simulink model "gm_sampleModel12940_sub"  (R2023b)
settings: Solver=VariableStepAuto  StartTime=0.0  StopTime=10.0  RelTol=1e-3
libraries: hdlsllib x3, simulink x2
(part 1 of 2)
settings Model: Creator=Tsmc  LastModifiedBy=Tsmc
settings OptimizationCC: BlockReduction=off  ConditionallyExecuteInputs=off
settings DebuggingCC: InheritedTsInSrcMsg=none

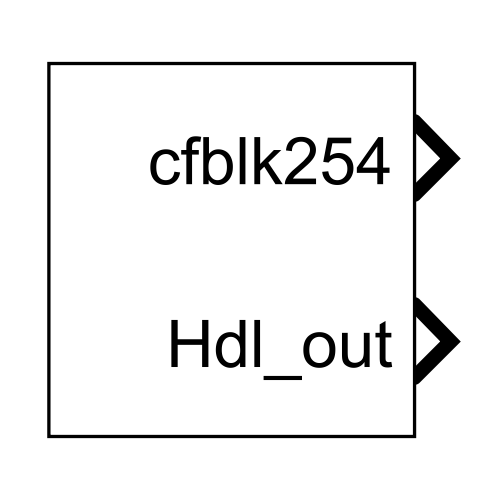
[thumbnail: Simulink's stored preview of the top-level diagram]
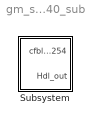
== system gm_sampleModel12940_sub ==
  Subsystem : Subsystem

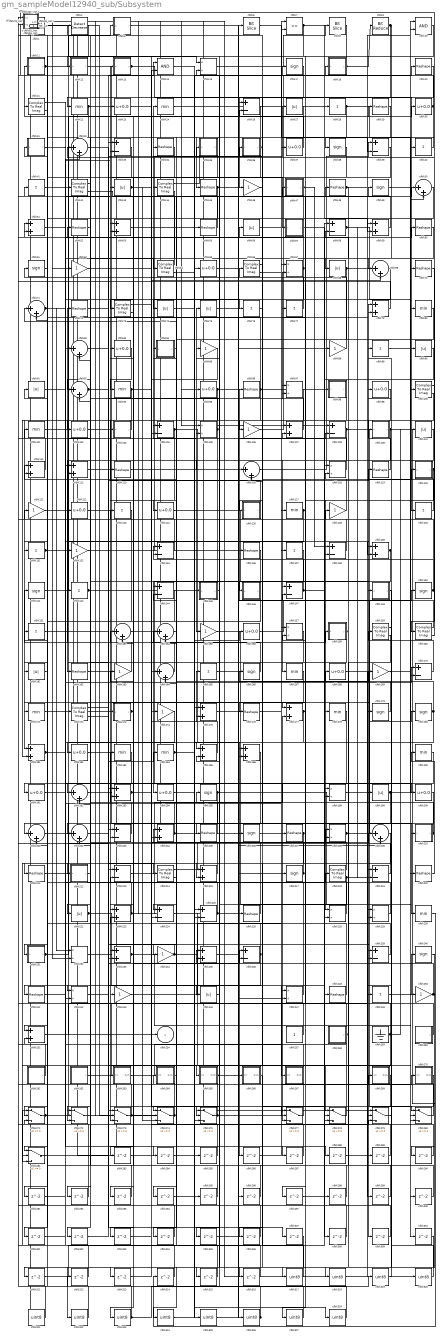
== system gm_sampleModel12940_sub/Subsystem ==
  cfblk1 : simulink/Logic and Bit Operations/Detect Decrease  vinit=0.0  OutDataTypeStr=uint8
      settings: LibrarySourceBlock=|
      | hdlsllib/Logic and Bit
      | Operations/Detect
      | Decrease
  cfblk10 : Logic  AllPortsSameDT=off  OutDataTypeStr=boolean
  cfblk{21,42,44,64,66,73,100,159..160,172,214,218} (12 alike) : ComplexToRealImag
  cfblk100_term0 : Terminator
  cfblk{22,24,80,93,101,127,167,171,178,183..184,190,230} (13 alike) : MinMax  OutDataTypeStr=uint8
  cfblk{23,30,37,65,83,95,99,102,122,124,156,168,182,191,194,200} (16 alike) : Bias  Bias=0.0  SaturateOnIntegerOverflow=off
  cfblk103 : Subsystem  mask(Real World Value Increment){}
      mask help: Simulink:masks:RealWorldValueIncrement_MD
      mask Display: disp('V++')
  cfblk{26,33,39,58,104,108,134,138,144,147,170,203,213,219,224..225,236,239} (18 alike) : Sum  Inputs=+-  OutDataTypeStr=uint8
  cfblk{15,67,97,105,118,157,198,208,228..229,232,242,247} (13 alike) : Product  Inputs=*/  OutDataTypeStr=uint8  RndMeth=Zero  SaturateOnIntegerOverflow=on
  cfblk{46,62,85,88,106,121,128,132,155,163,169,174,234,243,250} (15 alike) : Gain  OutDataTypeStr=uint8
  cfblk{51,53,59,79,107,111..112,139,175,177,181,185..186,193,204,215,223,233,235,251} (20 alike) : Sum  OutDataTypeStr=uint8
  cfblk109 : Subsystem  mask(Real World Value Increment){}
      mask help: Simulink:masks:RealWorldValueIncrement_MD
      mask Display: disp('V++')
  cfblk11 : Subsystem  mask(Compare To Zero){relop=<=, OutDataTypeStr=uint8, ZeroCross=on}
      mask prompts: relop "Simulink:masks:Operator_MP"; OutDataTypeStr "Simulink:masks:OutputDataType_MP"; ZeroCross "Simulink:masks:EnableZerocrossingDetection_MP"
      mask help: Simulink:masks:CompareToZero_MD
      mask init:
      | OutDataTypeStr = 'uint8';
      | ZeroCross = 'on';
      | blkName = 'sampleModel12940_sub/Subsystem/cfblk11';
      | relop = '<=';
      | setValue = 'fixdt(0, 8)';
      mask TypeOptions relop: == | ~= | < | <= | >= | >
      mask TypeOptions OutDataTypeStr: Simulink:masks:uint8 | Simulink:masks:boolean
      mask Callback ZeroCross: sl('zeroCrossEnable', gcbh);
      mask Display: disp([relop,' 0'])
  cfblk{27,43,56,68,74..75,90..91,110,161,199,222,245} (13 alike) : Abs  OutDataTypeStr=uint8  SaturateOnIntegerOverflow=off
  cfblk{20,29,34,45,48,52,55,60,70,72,96,113,119,136,162,176,205,207,211,220,226,241,248} (23 alike) : Reshape
  cfblk115_inst : Subsystem
  cfblk{32,50,69,71,82,92,116,153..154,164,192,201..202,209} (14 alike) : Sum  Inputs=|++  OutDataTypeStr=uint8
  cfblk12 : Subsystem  mask(Detect Rise Positive){vinit=double(0), InputProcessing=Elements as channels (sample based), OutDataTypeStr=uint8}
      mask prompts: vinit "Simulink:masks:InitialCondition_MP"; InputProcessing "Simulink:masks:InputProcessing_MP"; OutDataTypeStr "Simulink:masks:OutputDataType_MP"
      mask help: Simulink:masks:DetectRisePositive_MD
      mask init:
      | InputProcessing = 'Elements as channels (sample based)';
      | OutDataTypeStr = 'uint8';
      | vinit = double(0);
      mask TypeOptions InputProcessing: Simulink:masks:ColumnsAsChannelsFrameBased | Simulink:masks:ElementsAsChannelsSampleBased
      mask TypeOptions OutDataTypeStr: Simulink:masks:uint8 | Simulink:masks:boolean
      mask Display: fprintf('U > 0\n&  NOT\nU/z > 0')
  cfblk120 : Subsystem  mask(Real World Value Increment){}
      mask help: Simulink:masks:RealWorldValueIncrement_MD
      mask Display: disp('V++')
  cfblk{28,40..41,76..77,89,123,130..131,137,142,151,165,249} (14 alike) : Sum  Inputs=+  OutDataTypeStr=uint8
  cfblk126 : Subsystem  mask(Real World Value Increment){}
      mask help: Simulink:masks:RealWorldValueIncrement_MD
      mask Display: disp('V++')
  cfblk129_inst : Subsystem
  cfblk13 : Subsystem  mask(Compare To Zero){relop=<=, OutDataTypeStr=uint8, ZeroCross=on}
      mask prompts: relop "Simulink:masks:Operator_MP"; OutDataTypeStr "Simulink:masks:OutputDataType_MP"; ZeroCross "Simulink:masks:EnableZerocrossingDetection_MP"
      mask help: Simulink:masks:CompareToZero_MD
      mask init:
      | OutDataTypeStr = 'uint8';
      | ZeroCross = 'on';
      | blkName = 'sampleModel12940_sub/Subsystem/cfblk13';
      | relop = '<=';
      | setValue = 'fixdt(0, 8)';
      mask TypeOptions relop: == | ~= | < | <= | >= | >
      mask TypeOptions OutDataTypeStr: Simulink:masks:uint8 | Simulink:masks:boolean
      mask Callback ZeroCross: sl('zeroCrossEnable', gcbh);
      mask Display: disp([relop,' 0'])
  cfblk14 : Logic  AllPortsSameDT=off  OutDataTypeStr=boolean
  cfblk{17,38,49,61,141,150,166,179..180,195,206,217,240} (13 alike) : Signum
  cfblk145 : Subsystem  mask(Real World Value Increment){}
      mask help: Simulink:masks:RealWorldValueIncrement_MD
      mask Display: disp('V++')
  cfblk146 : Subsystem  mask(Real World Value Increment){}
      mask help: Simulink:masks:RealWorldValueIncrement_MD
      mask Display: disp('V++')
  cfblk148_inst : Subsystem
  cfblk149 : Subsystem  mask(Real World Value Increment){}
      mask help: Simulink:masks:RealWorldValueIncrement_MD
      mask Display: disp('V++')
  cfblk152_inst : Subsystem
  cfblk158 : Subsystem  mask(Real World Value Increment){}
      mask help: Simulink:masks:RealWorldValueIncrement_MD
      mask Display: disp('V++')
  cfblk16_inst : Subsystem
  cfblk173 : Subsystem  mask(Real World Value Increment){}
      mask help: Simulink:masks:RealWorldValueIncrement_MD
      mask Display: disp('V++')
  cfblk18 : Subsystem  mask(Real World Value Increment){}
      mask help: Simulink:masks:RealWorldValueIncrement_MD
      mask Display: disp('V++')
  cfblk19_inst : Subsystem
  cfblk2 : simulink/Logic and Bit Operations/Detect Decrease  vinit=0.0  OutDataTypeStr=uint8
      settings: LibrarySourceBlock=|
      | hdlsllib/Logic and Bit
      | Operations/Detect
      | Decrease
  cfblk210 : Subsystem  mask(Real World Value Increment){}
      mask help: Simulink:masks:RealWorldValueIncrement_MD
      mask Display: disp('V++')
  cfblk212 : Subsystem  mask(Real World Value Increment){}
      mask help: Simulink:masks:RealWorldValueIncrement_MD
      mask Display: disp('V++')
  cfblk216_inst : Subsystem
  cfblk21_term1 : Terminator
  cfblk221_inst : Subsystem
  cfblk231 : Subsystem  mask(Real World Value Increment){}
      mask help: Simulink:masks:RealWorldValueIncrement_MD
      mask Display: disp('V++')
  cfblk257 : Constant  OutDataTypeStr=uint8  SampleTime=-1
  cfblk258 : Subsystem  mask(Counter Limited){uplimit=double(7), tsamp=double(-1)}
      mask prompts: uplimit "Simulink:masks:UpperLimit_MP"; tsamp "Simulink:masks:SampleTime_MP"
      mask help: Simulink:masks:CounterLimited_MD
      mask init:
      | nbits = double(8);
      | tsamp = double(-1);
      | uplimit = double(7);
  cfblk259 : Ground
  cfblk260 : Subsystem  mask(Counter Free-Running){NumBits=double(16), tsamp=double(-1)}
      mask prompts: NumBits "Simulink:masks:NumberOfBits_MP"; tsamp "Simulink:masks:SampleTime_MP"
      mask help: Simulink:masks:CounterFreeRunning_MD
  cfblk261 : Subsystem  mask(Counter Limited){uplimit=double(7), tsamp=double(-1)}
      mask prompts: uplimit "Simulink:masks:UpperLimit_MP"; tsamp "Simulink:masks:SampleTime_MP"
      mask help: Simulink:masks:CounterLimited_MD
      mask init:
      | nbits = double(8);
      | tsamp = double(-1);
      | uplimit = double(7);
  cfblk262 : Subsystem  mask(Counter Limited){uplimit=double(7), tsamp=double(-1)}
      mask prompts: uplimit "Simulink:masks:UpperLimit_MP"; tsamp "Simulink:masks:SampleTime_MP"
      mask help: Simulink:masks:CounterLimited_MD
      mask init:
      | nbits = double(8);
      | tsamp = double(-1);
      | uplimit = double(7);
  cfblk263 : Subsystem
  cfblk264 : Subsystem
  cfblk265 : Subsystem
  cfblk266 : Subsystem
  cfblk267 : Subsystem
  cfblk269 : Subsystem
  cfblk270 : Subsystem
  cfblk{271..275,277..281} (10 alike) : Switch  OutDataTypeStr=uint8  SaturateOnIntegerOverflow=off  InputSameDT=off
  cfblk{283..316} (34 alike) : Delay  SampleTime=1
  cfblk3 : Subsystem  mask(Detect Fall Nonpositive){vinit=double(0), InputProcessing=Elements as channels (sample based), OutDataTypeStr=uint8}
      mask prompts: vinit "Simulink:masks:InitialCondition_MP"; InputProcessing "Simulink:masks:InputProcessing_MP"; OutDataTypeStr "Simulink:masks:OutputDataType_MP"
      mask help: Simulink:masks:DetectFallNonpositive_MD
      mask init:
      | InputProcessing = 'Elements as channels (sample based)';
      | OutDataTypeStr = 'uint8';
      | vinit = double(0);
      mask TypeOptions InputProcessing: Simulink:masks:ColumnsAsChannelsFrameBased | Simulink:masks:ElementsAsChannelsSampleBased
      mask TypeOptions OutDataTypeStr: Simulink:masks:uint8 | Simulink:masks:boolean
      mask Display: fprintf('U <= 0\n&  NOT\nU/z <= 0')
  cfblk31 : Subsystem  mask(Real World Value Increment){}
      mask help: Simulink:masks:RealWorldValueIncrement_MD
      mask Display: disp('V++')
  cfblk{317..328} (12 alike) : DataTypeConversion  OutDataTypeStr=uint8  SaturateOnIntegerOverflow=off  RndMeth=Floor
  cfblk35 : Subsystem  mask(Real World Value Increment){}
      mask help: Simulink:masks:RealWorldValueIncrement_MD
      mask Display: disp('V++')
  cfblk36 : Subsystem  mask(Real World Value Increment){}
      mask help: Simulink:masks:RealWorldValueIncrement_MD
      mask Display: disp('V++')
  cfblk47 : Subsystem  mask(Real World Value Increment){}
      mask help: Simulink:masks:RealWorldValueIncrement_MD
      mask Display: disp('V++')
  cfblk57 : Subsystem  mask(Real World Value Increment){}
      mask help: Simulink:masks:RealWorldValueIncrement_MD
      mask Display: disp('V++')
  cfblk6 : hdlsllib/Logic and Bit Operations/Bit Slice  lidx=7  ridx=0
  cfblk63_inst : Subsystem
  cfblk7 : RelationalOperator  Operator=<=  OutDataTypeStr=boolean  InputSameDT=off
  cfblk78_inst : Subsystem
  cfblk8 : hdlsllib/Logic and Bit Operations/Bit Slice  lidx=7  ridx=0
  cfblk81_inst : Subsystem
  cfblk84 : Subsystem  mask(Real World Value Increment){}
      mask help: Simulink:masks:RealWorldValueIncrement_MD
      mask Display: disp('V++')
  cfblk9 : hdlsllib/Logic and Bit Operations/Bit Reduce  mode=AND
  cfblk94_inst : Subsystem
  cfblk98 : Subsystem  mask(Real World Value Increment){}
      mask help: Simulink:masks:RealWorldValueIncrement_MD
      mask Display: disp('V++')
  cfblk254 : Outport  OutDataTypeStr=uint8  SampleTime=1  VectorParamsAs1DForOutWhenUnconnected=off
  Hdl_out : Outport  Port=2  OutDataTypeStr=uint8  SampleTime=1
  wires:
  cfblk1/1 -> cfblk15/1
  cfblk10/1 -> cfblk273/3
  cfblk100/1 -> cfblk100_term0/1
  cfblk100/2 -> cfblk309/1
  cfblk101/1 -> cfblk185/1
  cfblk102/1 -> cfblk273/2
  cfblk103/1(y) -> cfblk181/1
  cfblk104/1 -> cfblk203/2, cfblk286/1
  cfblk105/1 -> cfblk216_inst/2(in2), cfblk194/1
  cfblk106/1 -> cfblk20/1
  cfblk107/1 -> cfblk67/2
  cfblk108/1 -> cfblk280/1, cfblk167/1
  cfblk109/1(y) -> cfblk311/1, cfblk155/1
  cfblk11/1(y) -> cfblk3/1(U), cfblk254/1
  cfblk110/1 -> cfblk162/1
  cfblk111/1 -> cfblk19_inst/1(in1)
  cfblk112/1 -> cfblk296/1
  cfblk113/1 -> cfblk75/1
  cfblk115_inst/1(out1) -> cfblk320/1
  cfblk116/1 -> cfblk39/1
  cfblk118/1 -> cfblk24/1
  cfblk119/1 -> cfblk79/1
  cfblk12/1(Y) -> cfblk277/3
  cfblk120/1(y) -> cfblk277/1, cfblk228/1, cfblk228/2, cfblk229/2
  cfblk121/1 -> cfblk273/1
  cfblk122/1 -> cfblk230/1
  cfblk123/1 -> cfblk281/1
  cfblk124/1 -> cfblk149/1(u)
  cfblk126/1(y) -> cfblk13/1(u)
  cfblk127/1 -> cfblk275/2, cfblk182/1, cfblk177/1, cfblk305/1
  cfblk128/1 -> cfblk34/1
  cfblk129_inst/1(out1) -> cfblk279/1, cfblk285/1, cfblk173/1(u)
  cfblk13/1(y) -> cfblk46/1, cfblk130/1
  cfblk130/1 -> cfblk16_inst/1(in1)
  cfblk131/1 -> cfblk26/2, cfblk172/1
  cfblk132/1 -> cfblk6/1
  cfblk134/1 -> cfblk123/1
  cfblk136/1 -> cfblk293/1
  cfblk137/1 -> cfblk283/1
  cfblk138/1 -> cfblk221_inst/1(in1)
  cfblk139/1 -> cfblk205/1, cfblk292/1
  cfblk14/1 -> cfblk295/1
  cfblk141/1 -> cfblk105/2
  cfblk142/1 -> cfblk82/2, cfblk147/1, cfblk229/1
  cfblk144/1 -> cfblk271/2
  cfblk145/1(y) -> cfblk95/1
  cfblk146/1(y) -> cfblk302/1
  cfblk147/1 -> cfblk278/3, cfblk85/1
  cfblk148_inst/1(out1) -> cfblk98/1(u)
  cfblk149/1(y) -> cfblk249/1
  cfblk15/1 -> cfblk8/1
  cfblk150/1 -> cfblk134/1, cfblk128/1
  cfblk151/1 -> cfblk213/1
  cfblk152_inst/1(out1) -> cfblk226/1, cfblk232/2
  cfblk153/1 -> cfblk247/1
  cfblk154/1 -> cfblk84/1(u)
  cfblk155/1 -> cfblk310/1
  cfblk156/1 -> cfblk100/1
  cfblk157/1 -> cfblk303/1
  cfblk158/1(y) -> cfblk297/1, cfblk242/1
  cfblk159/1 -> cfblk317/1
  cfblk159/2 -> cfblk318/1
  cfblk16_inst/1(out1) -> cfblk274/2
  cfblk160/1 -> cfblk96/1
  cfblk160/2 -> cfblk32/1
  cfblk161/1 -> cfblk71/2
  cfblk162/1 -> cfblk219/1
  cfblk163/1 -> cfblk141/1
  cfblk164/1 -> cfblk72/1
  cfblk165/1 -> cfblk210/1(u)
  cfblk166/1 -> cfblk153/1
  cfblk167/1 -> cfblk251/1
  cfblk168/1 -> cfblk289/1
  cfblk169/1 -> cfblk70/1
  cfblk17/1 -> cfblk206/1
  cfblk170/1 -> cfblk99/1
  cfblk171/1 -> cfblk82/1
  cfblk172/1 -> cfblk265/1(In1)
  cfblk172/2 -> cfblk14/1
  cfblk173/1(y) -> cfblk53/1, cfblk153/2
  cfblk174/1 -> cfblk242/2
  cfblk175/1 -> cfblk248/1
  cfblk176/1 -> cfblk168/1
  cfblk177/1 -> cfblk186/2, cfblk157/2, cfblk77/1
  cfblk178/1 -> cfblk198/1
  cfblk179/1 -> cfblk71/1
  cfblk18/1(y) -> cfblk9/1, cfblk12/1(U)
  cfblk180/1 -> cfblk66/1, cfblk275/3
  cfblk181/1 -> cfblk32/2, cfblk170/1
  cfblk182/1 -> cfblk325/1
  cfblk183/1 -> cfblk291/1
  cfblk184/1 -> cfblk49/1, cfblk156/1
  cfblk185/1 -> cfblk165/1
  cfblk186/1 -> cfblk304/1
  cfblk19_inst/1(out1) -> cfblk42/1, cfblk207/1, cfblk28/1
  cfblk190/1 -> cfblk192/1
  cfblk191/1 -> cfblk43/1
  cfblk192/1 -> cfblk225/1
  cfblk193/1 -> cfblk116/1, cfblk158/1(u)
  cfblk194/1 -> cfblk65/1
  cfblk195/1 -> cfblk280/3, cfblk243/1
  cfblk198/1 -> cfblk80/1
  cfblk199/1 -> cfblk50/2, cfblk272/3
  cfblk2/1 -> cfblk301/1
  cfblk20/1 -> cfblk22/1
  cfblk200/1 -> cfblk215/2
  cfblk201/1 -> cfblk105/1
  cfblk202/1 -> cfblk239/1
  cfblk203/1 -> cfblk121/1
  cfblk204/1 -> cfblk239/2, cfblk111/1
  cfblk205/1 -> cfblk183/1
  cfblk206/1 -> cfblk7/2
  cfblk207/1 -> cfblk281/2, cfblk223/1, cfblk266/1(In1)
  cfblk208/1 -> cfblk180/1, cfblk10/2
  cfblk209/1 -> cfblk323/1
  cfblk21/1 -> cfblk287/1
  cfblk21/2 -> cfblk21_term1/1
  cfblk210/1(y) -> cfblk52/1, cfblk193/2
  cfblk211/1 -> cfblk203/1
  cfblk212/1(y) -> cfblk92/2
  cfblk213/1 -> cfblk177/2
  cfblk214/1 -> cfblk127/1
  cfblk214/2 -> cfblk112/2
  cfblk215/1 -> cfblk129_inst/1(in1)
  cfblk216_inst/1(out1) -> cfblk136/1
  cfblk217/1 -> cfblk166/1, cfblk101/1
  cfblk218/1 -> cfblk83/1
  cfblk218/2 -> cfblk59/1, cfblk315/1, cfblk120/1(u)
  cfblk219/1 -> cfblk152_inst/1(in1)
  cfblk22/1 -> cfblk211/1, cfblk57/1(u)
  cfblk220/1 -> cfblk190/1
  cfblk221_inst/1(out1) -> cfblk108/1, cfblk62/1
  cfblk222/1 -> cfblk308/1, cfblk184/1
  cfblk223/1 -> cfblk213/2, cfblk67/1
  cfblk224/1 -> cfblk278/1
  cfblk225/1 -> cfblk150/1, cfblk113/1
  cfblk226/1 -> cfblk185/2
  cfblk228/1 -> cfblk122/1
  cfblk229/1 -> cfblk31/1(u)
  cfblk23/1 -> cfblk278/2
  cfblk230/1 -> cfblk314/1
  cfblk231/1(y) -> cfblk164/1, cfblk157/1
  cfblk232/1 -> cfblk267/1(In1)
  cfblk233/1 -> cfblk280/2, cfblk299/1, cfblk298/1
  cfblk234/1 -> cfblk233/1, cfblk300/1
  cfblk235/1 -> cfblk326/1
  cfblk236/1 -> cfblk241/1, cfblk223/2
  cfblk239/1 -> cfblk118/2
  cfblk24/1 -> cfblk175/1
  cfblk240/1 -> cfblk290/1
  cfblk241/1 -> cfblk218/1
  cfblk242/1 -> cfblk97/1
  cfblk243/1 -> cfblk107/1
  cfblk245/1 -> cfblk195/1
  cfblk247/1 -> cfblk44/1
  cfblk248/1 -> cfblk91/1
  cfblk249/1 -> cfblk240/1
  cfblk250/1 -> cfblk163/1, cfblk47/1(u)
  cfblk251/1 -> cfblk208/1
  cfblk257/1 -> cfblk36/1(u)
  cfblk258/1(y) -> cfblk147/2, cfblk118/1
  cfblk259/1 -> cfblk281/3, cfblk221_inst/2(in2), cfblk164/2, cfblk110/1
  cfblk26/1 -> cfblk74/1
  cfblk260/1(y) -> cfblk151/1
  cfblk261/1(y) -> cfblk16_inst/2(in2)
  cfblk262/1(y) -> cfblk179/1
  cfblk263/1(Out1) -> cfblk137/1
  cfblk264/1(Out1) -> cfblk154/1
  cfblk265/1(Out1) -> cfblk107/2, cfblk288/1, cfblk169/1
  cfblk266/1(Out1) -> cfblk316/1
  cfblk267/1(Out1) -> cfblk26/1
  cfblk269/1(Out1) -> cfblk279/2
  cfblk27/1 -> cfblk231/1(u)
  cfblk270/1(Out1) -> cfblk306/1
  cfblk271/1 -> cfblk58/1, cfblk233/2
  cfblk272/1 -> cfblk236/1
  cfblk273/1 -> cfblk78_inst/2(in2), cfblk55/1
  cfblk274/1 -> cfblk51/1, Hdl_out/1
  cfblk275/1 -> cfblk186/1, cfblk134/2, cfblk270/1(In1)
  cfblk277/1 -> cfblk23/1
  cfblk278/1 -> cfblk112/1
  cfblk279/1 -> cfblk89/1
  cfblk28/1 -> cfblk272/1, cfblk250/1
  cfblk280/1 -> cfblk264/1(In1)
  cfblk281/1 -> cfblk119/1
  cfblk283/1 -> cfblk1/1
  cfblk284/1 -> cfblk328/1
  cfblk285/1 -> cfblk202/2
  cfblk286/1 -> cfblk7/1
  cfblk287/1 -> cfblk63_inst/1(in1)
  cfblk288/1 -> cfblk50/1
  cfblk289/1 -> cfblk81_inst/2(in2)
  cfblk29/1 -> cfblk126/1(u)
  cfblk290/1 -> cfblk144/2
  cfblk291/1 -> cfblk193/1
  cfblk292/1 -> cfblk19_inst/2(in2)
  cfblk293/1 -> cfblk192/2
  cfblk294/1 -> cfblk97/2
  cfblk295/1 -> cfblk251/2
  cfblk296/1 -> cfblk111/2
  cfblk297/1 -> cfblk208/2
  cfblk298/1 -> cfblk53/2
  cfblk299/1 -> cfblk58/2
  cfblk3/1(Y) -> cfblk217/1
  cfblk30/1 -> cfblk81_inst/1(in1), cfblk45/1
  cfblk300/1 -> cfblk15/2
  cfblk301/1 -> cfblk33/2
  cfblk302/1 -> cfblk215/1
  cfblk303/1 -> cfblk175/2
  cfblk304/1 -> cfblk271/3
  cfblk305/1 -> cfblk108/2
  cfblk306/1 -> cfblk94_inst/2(in2)
  cfblk307/1 -> cfblk324/1
  cfblk308/1 -> cfblk104/1
  cfblk309/1 -> cfblk129_inst/2(in2)
  cfblk31/1(y) -> cfblk76/1
  cfblk310/1 -> cfblk322/1
  cfblk311/1 -> cfblk138/2
  cfblk312/1 -> cfblk78_inst/1(in1)
  cfblk313/1 -> cfblk279/3
  cfblk314/1 -> cfblk271/1
  cfblk315/1 -> cfblk272/2
  cfblk316/1 -> cfblk204/1
  cfblk317/1 -> cfblk56/1
  cfblk318/1 -> cfblk109/1(u)
  cfblk319/1 -> cfblk159/1
  cfblk32/1 -> cfblk245/1
  cfblk320/1 -> cfblk269/1(In1)
  cfblk321/1 -> cfblk115_inst/1(in1)
  cfblk322/1 -> cfblk115_inst/2(in2)
  cfblk323/1 -> cfblk319/1, cfblk312/1
  cfblk324/1 -> cfblk209/1
  cfblk325/1 -> cfblk209/2
  cfblk326/1 -> cfblk63_inst/2(in2), cfblk51/2
  cfblk327/1 -> cfblk235/1
  cfblk328/1 -> cfblk235/2
  cfblk33/1 -> cfblk92/1
  cfblk34/1 -> cfblk313/1
  cfblk35/1(y) -> cfblk191/1
  cfblk36/1(y) -> cfblk73/1, cfblk225/2
  cfblk37/1 -> cfblk11/1(u)
  cfblk38/1 -> cfblk275/1
  cfblk39/1 -> cfblk263/1(In1)
  cfblk40/1 -> cfblk38/1
  cfblk41/1 -> cfblk64/1
  cfblk42/1 -> cfblk102/1
  cfblk42/2 -> cfblk48/1
  cfblk43/1 -> cfblk69/2, cfblk274/3
  cfblk44/1 -> cfblk27/1
  cfblk44/2 -> cfblk222/1
  cfblk45/1 -> cfblk212/1(u), cfblk247/2
  cfblk46/1 -> cfblk146/1(u)
  cfblk47/1(y) -> cfblk274/1, cfblk138/1
  cfblk48/1 -> cfblk68/1, cfblk10/1
  cfblk49/1 -> cfblk40/1
  cfblk50/1 -> cfblk161/1
  cfblk51/1 -> cfblk284/1
  cfblk52/1 -> cfblk132/1
  cfblk53/1 -> cfblk17/1
  cfblk55/1 -> cfblk21/1
  cfblk56/1 -> cfblk37/1
  cfblk57/1(y) -> cfblk178/1
  cfblk58/1 -> cfblk90/1, cfblk30/1, cfblk219/2
  cfblk59/1 -> cfblk216_inst/1(in1)
  cfblk6/1 -> cfblk39/2
  cfblk60/1 -> cfblk202/1
  cfblk61/1 -> cfblk201/2
  cfblk62/1 -> cfblk14/2
  cfblk63_inst/1(out1) -> cfblk145/1(u)
  cfblk64/1 -> cfblk2/1
  cfblk64/2 -> cfblk29/1
  cfblk65/1 -> cfblk139/1
  cfblk66/1 -> cfblk171/1
  cfblk66/2 -> cfblk18/1(u)
  cfblk67/1 -> cfblk176/1, cfblk148_inst/2(in2)
  cfblk68/1 -> cfblk170/2, cfblk154/2
  cfblk69/1 -> cfblk234/1
  cfblk7/1 -> cfblk59/2, cfblk104/2
  cfblk70/1 -> cfblk160/1
  cfblk71/1 -> cfblk60/1, cfblk139/2, cfblk232/1
  cfblk72/1 -> cfblk307/1
  cfblk73/1 -> cfblk174/1
  cfblk73/2 -> cfblk61/1
  cfblk74/1 -> cfblk277/2
  cfblk75/1 -> cfblk88/1
  cfblk76/1 -> cfblk116/2
  cfblk77/1 -> cfblk41/1
  cfblk78_inst/1(out1) -> cfblk321/1
  cfblk79/1 -> cfblk152_inst/2(in2)
  cfblk8/1 -> cfblk327/1
  cfblk80/1 -> cfblk224/1
  cfblk81_inst/1(out1) -> cfblk94_inst/1(in1)
  cfblk82/1 -> cfblk199/1
  cfblk83/1 -> cfblk93/1
  cfblk84/1(y) -> cfblk294/1
  cfblk85/1 -> cfblk204/2
  cfblk88/1 -> cfblk33/1
  cfblk89/1 -> cfblk220/1
  cfblk9/1 -> cfblk69/1, cfblk106/1
  cfblk90/1 -> cfblk198/2
  cfblk91/1 -> cfblk200/1
  cfblk92/1 -> cfblk79/2, cfblk214/1, cfblk35/1(u)
  cfblk93/1 -> cfblk224/2, cfblk103/1(u)
  cfblk94_inst/1(out1) -> cfblk142/1
  cfblk95/1 -> cfblk236/2, cfblk144/1
  cfblk96/1 -> cfblk181/2, cfblk148_inst/1(in1)
  cfblk97/1 -> cfblk131/1
  cfblk98/1(y) -> cfblk124/1
  cfblk99/1 -> cfblk201/1

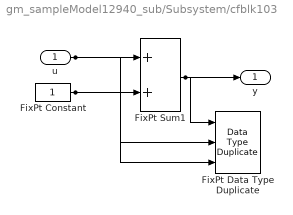
== system gm_sampleModel12940_sub/Subsystem/cfblk103 ==
  u : Inport  OutDataTypeStr=uint8  SampleTime=1
  FixPt Constant : Constant  DisableCoverage=on  OutDataTypeStr=Inherit: Inherit via back propagation  SampleTime=-1
  FixPt Data Type Duplicate : DataTypeDuplicate  DisableCoverage=on  NumInputPorts=3
  FixPt Sum1 : Sum  OutDataTypeStr=Inherit: Inherit via back propagation  InputSameDT=on  LockScale=on
  y : Outport  SampleTime=1
  wires:
  u/1 -> FixPt Sum1/1, FixPt Data Type Duplicate/2
  FixPt Constant/1 -> FixPt Sum1/2, FixPt Data Type Duplicate/3
  FixPt Sum1/1 -> FixPt Data Type Duplicate/1, y/1

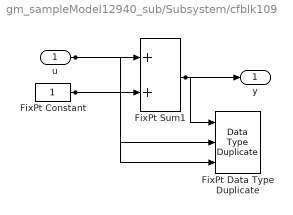
== system gm_sampleModel12940_sub/Subsystem/cfblk109 ==
  u : Inport  OutDataTypeStr=uint8  SampleTime=1
  FixPt Constant : Constant  DisableCoverage=on  OutDataTypeStr=Inherit: Inherit via back propagation  SampleTime=-1
  FixPt Data Type Duplicate : DataTypeDuplicate  DisableCoverage=on  NumInputPorts=3
  FixPt Sum1 : Sum  OutDataTypeStr=Inherit: Inherit via back propagation  InputSameDT=on  LockScale=on
  y : Outport  SampleTime=1
  wires:
  u/1 -> FixPt Sum1/1, FixPt Data Type Duplicate/2
  FixPt Constant/1 -> FixPt Sum1/2, FixPt Data Type Duplicate/3
  FixPt Sum1/1 -> FixPt Data Type Duplicate/1, y/1

== system gm_sampleModel12940_sub/Subsystem/cfblk11 ==
  u : Inport  OutDataTypeStr=uint8  SampleTime=1
  Compare : RelationalOperator  Operator=<=  OutDataTypeStr=fixdt(0, 8)
  Constant : Constant  DisableCoverage=on  Value=0  OutDataTypeStr=Inherit: Inherit via back propagation  SampleTime=-1  PreserveConstantTs=on
  y : Outport  SampleTime=1
  wires:
  u/1 -> Compare/1
  Compare/1 -> y/1
  Constant/1 -> Compare/2

== system gm_sampleModel12940_sub/Subsystem/cfblk115_inst ==
  in1 : Inport  OutDataTypeStr=uint8  SampleTime=1
  in2 : Inport  Port=2  OutDataTypeStr=uint8  SampleTime=1
  mul_cfblk115_dotp_mulcomp : Product  Inputs=**  OutDataTypeStr=uint8  SampleTime=1
  out1 : Outport  OutDataTypeStr=uint8  SampleTime=1
  wires:
  in1/1 -> mul_cfblk115_dotp_mulcomp/1
  in2/1 -> mul_cfblk115_dotp_mulcomp/2
  mul_cfblk115_dotp_mulcomp/1 -> out1/1

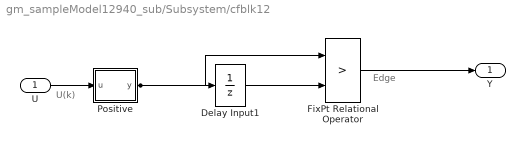
== system gm_sampleModel12940_sub/Subsystem/cfblk12 ==
  note: U(k)
  note: Edge
  U : Inport  OutDataTypeStr=uint8  SampleTime=1
  Delay Input1 : UnitDelay  Description=Store in Global RAM  DisableCoverage=on  InitialCondition=vinit  SampleTime=-1  HasFrameUpgradeWarning=on
  FixPt Relational Operator : RelationalOperator  Operator=>  OutDataTypeStr=fixdt(0, 8)  ZeroCross=off  InputSameDT=off
  Positive : Subsystem  mask(Compare To Zero){relop=>, OutDataTypeStr=boolean, ZeroCross=off}
      mask prompts: relop "Simulink:masks:Operator_MP"; OutDataTypeStr "Simulink:masks:OutputDataType_MP"; ZeroCross "Simulink:masks:EnableZerocrossingDetection_MP"
      mask help: Simulink:masks:CompareToZero_MD
      mask init:
      | OutDataTypeStr = 'boolean';
      | ZeroCross = 'off';
      | blkName = 'sampleModel12940_sub/Subsystem/cfblk12/Positive';
      | relop = '>';
      | setValue = 'boolean';
      mask TypeOptions relop: == | ~= | < | <= | >= | >
      mask TypeOptions OutDataTypeStr: Simulink:masks:uint8 | Simulink:masks:boolean
      mask Callback ZeroCross: sl('zeroCrossEnable', gcbh);
      mask Display: disp([relop,' 0'])
  Y : Outport  SampleTime=1
  wires:
  U/1 -> Positive/1(u)
  Delay Input1/1 -> FixPt Relational Operator/2
  FixPt Relational Operator/1 -> Y/1
  Positive/1(y) -> FixPt Relational Operator/1, Delay Input1/1

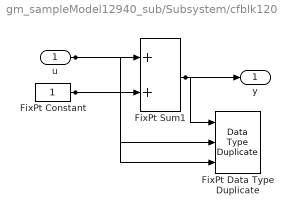
== system gm_sampleModel12940_sub/Subsystem/cfblk120 ==
  u : Inport  OutDataTypeStr=uint8  SampleTime=1
  FixPt Constant : Constant  DisableCoverage=on  OutDataTypeStr=Inherit: Inherit via back propagation  SampleTime=-1
  FixPt Data Type Duplicate : DataTypeDuplicate  DisableCoverage=on  NumInputPorts=3
  FixPt Sum1 : Sum  OutDataTypeStr=Inherit: Inherit via back propagation  InputSameDT=on  LockScale=on
  y : Outport  SampleTime=1
  wires:
  u/1 -> FixPt Sum1/1, FixPt Data Type Duplicate/2
  FixPt Constant/1 -> FixPt Sum1/2, FixPt Data Type Duplicate/3
  FixPt Sum1/1 -> FixPt Data Type Duplicate/1, y/1

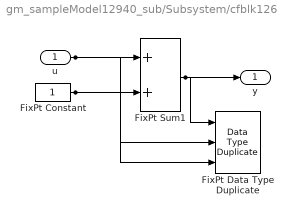
== system gm_sampleModel12940_sub/Subsystem/cfblk126 ==
  u : Inport  OutDataTypeStr=uint8  SampleTime=1
  FixPt Constant : Constant  DisableCoverage=on  OutDataTypeStr=Inherit: Inherit via back propagation  SampleTime=-1
  FixPt Data Type Duplicate : DataTypeDuplicate  DisableCoverage=on  NumInputPorts=3
  FixPt Sum1 : Sum  OutDataTypeStr=Inherit: Inherit via back propagation  InputSameDT=on  LockScale=on
  y : Outport  SampleTime=1
  wires:
  u/1 -> FixPt Sum1/1, FixPt Data Type Duplicate/2
  FixPt Constant/1 -> FixPt Sum1/2, FixPt Data Type Duplicate/3
  FixPt Sum1/1 -> FixPt Data Type Duplicate/1, y/1

== system gm_sampleModel12940_sub/Subsystem/cfblk129_inst ==
  in1 : Inport  OutDataTypeStr=uint8  SampleTime=1
  in2 : Inport  Port=2  OutDataTypeStr=uint8  SampleTime=1
  mul_cfblk129_dotp_mulcomp : Product  Inputs=**  OutDataTypeStr=uint8  SampleTime=1
  out1 : Outport  OutDataTypeStr=uint8  SampleTime=1
  wires:
  in1/1 -> mul_cfblk129_dotp_mulcomp/1
  in2/1 -> mul_cfblk129_dotp_mulcomp/2
  mul_cfblk129_dotp_mulcomp/1 -> out1/1

== system gm_sampleModel12940_sub/Subsystem/cfblk13 ==
  u : Inport  OutDataTypeStr=uint8  SampleTime=1
  Compare : RelationalOperator  Operator=<=  OutDataTypeStr=fixdt(0, 8)
  Constant : Constant  DisableCoverage=on  Value=0  OutDataTypeStr=Inherit: Inherit via back propagation  SampleTime=-1  PreserveConstantTs=on
  y : Outport  SampleTime=1
  wires:
  u/1 -> Compare/1
  Compare/1 -> y/1
  Constant/1 -> Compare/2

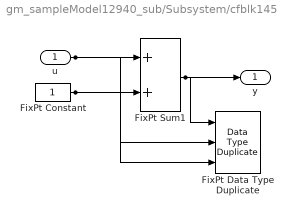
== system gm_sampleModel12940_sub/Subsystem/cfblk145 ==
  u : Inport  OutDataTypeStr=uint8  SampleTime=1
  FixPt Constant : Constant  DisableCoverage=on  OutDataTypeStr=Inherit: Inherit via back propagation  SampleTime=-1
  FixPt Data Type Duplicate : DataTypeDuplicate  DisableCoverage=on  NumInputPorts=3
  FixPt Sum1 : Sum  OutDataTypeStr=Inherit: Inherit via back propagation  InputSameDT=on  LockScale=on
  y : Outport  SampleTime=1
  wires:
  u/1 -> FixPt Sum1/1, FixPt Data Type Duplicate/2
  FixPt Constant/1 -> FixPt Sum1/2, FixPt Data Type Duplicate/3
  FixPt Sum1/1 -> FixPt Data Type Duplicate/1, y/1

== system gm_sampleModel12940_sub/Subsystem/cfblk146 ==
  u : Inport  OutDataTypeStr=uint8  SampleTime=1
  FixPt Constant : Constant  DisableCoverage=on  OutDataTypeStr=Inherit: Inherit via back propagation  SampleTime=-1
  FixPt Data Type Duplicate : DataTypeDuplicate  DisableCoverage=on  NumInputPorts=3
  FixPt Sum1 : Sum  OutDataTypeStr=Inherit: Inherit via back propagation  InputSameDT=on  LockScale=on
  y : Outport  SampleTime=1
  wires:
  u/1 -> FixPt Sum1/1, FixPt Data Type Duplicate/2
  FixPt Constant/1 -> FixPt Sum1/2, FixPt Data Type Duplicate/3
  FixPt Sum1/1 -> FixPt Data Type Duplicate/1, y/1

== system gm_sampleModel12940_sub/Subsystem/cfblk148_inst ==
  in1 : Inport  OutDataTypeStr=uint8  SampleTime=1
  in2 : Inport  Port=2  OutDataTypeStr=uint8  SampleTime=1
  mul_cfblk148_dotp_mulcomp : Product  Inputs=**  OutDataTypeStr=uint8  SampleTime=1
  out1 : Outport  OutDataTypeStr=uint8  SampleTime=1
  wires:
  in1/1 -> mul_cfblk148_dotp_mulcomp/1
  in2/1 -> mul_cfblk148_dotp_mulcomp/2
  mul_cfblk148_dotp_mulcomp/1 -> out1/1

== system gm_sampleModel12940_sub/Subsystem/cfblk149 ==
  u : Inport  OutDataTypeStr=uint8  SampleTime=1
  FixPt Constant : Constant  DisableCoverage=on  OutDataTypeStr=Inherit: Inherit via back propagation  SampleTime=-1
  FixPt Data Type Duplicate : DataTypeDuplicate  DisableCoverage=on  NumInputPorts=3
  FixPt Sum1 : Sum  OutDataTypeStr=Inherit: Inherit via back propagation  InputSameDT=on  LockScale=on
  y : Outport  SampleTime=1
  wires:
  u/1 -> FixPt Sum1/1, FixPt Data Type Duplicate/2
  FixPt Constant/1 -> FixPt Sum1/2, FixPt Data Type Duplicate/3
  FixPt Sum1/1 -> FixPt Data Type Duplicate/1, y/1

== system gm_sampleModel12940_sub/Subsystem/cfblk152_inst ==
  in1 : Inport  OutDataTypeStr=uint8  SampleTime=1
  in2 : Inport  Port=2  OutDataTypeStr=uint8  SampleTime=1
  mul_cfblk152_dotp_mulcomp : Product  Inputs=**  OutDataTypeStr=uint8  SampleTime=1
  out1 : Outport  OutDataTypeStr=uint8  SampleTime=1
  wires:
  in1/1 -> mul_cfblk152_dotp_mulcomp/1
  in2/1 -> mul_cfblk152_dotp_mulcomp/2
  mul_cfblk152_dotp_mulcomp/1 -> out1/1

== system gm_sampleModel12940_sub/Subsystem/cfblk158 ==
  u : Inport  OutDataTypeStr=uint8  SampleTime=1
  FixPt Constant : Constant  DisableCoverage=on  OutDataTypeStr=Inherit: Inherit via back propagation  SampleTime=-1
  FixPt Data Type Duplicate : DataTypeDuplicate  DisableCoverage=on  NumInputPorts=3
  FixPt Sum1 : Sum  OutDataTypeStr=Inherit: Inherit via back propagation  InputSameDT=on  LockScale=on
  y : Outport  SampleTime=1
  wires:
  u/1 -> FixPt Sum1/1, FixPt Data Type Duplicate/2
  FixPt Constant/1 -> FixPt Sum1/2, FixPt Data Type Duplicate/3
  FixPt Sum1/1 -> FixPt Data Type Duplicate/1, y/1

== system gm_sampleModel12940_sub/Subsystem/cfblk16_inst ==
  in1 : Inport  OutDataTypeStr=uint8  SampleTime=1
  in2 : Inport  Port=2  OutDataTypeStr=uint8  SampleTime=1
  mul_cfblk16_dotp_mulcomp : Product  Inputs=**  OutDataTypeStr=uint8  SampleTime=1
  out1 : Outport  OutDataTypeStr=uint8  SampleTime=1
  wires:
  in1/1 -> mul_cfblk16_dotp_mulcomp/1
  in2/1 -> mul_cfblk16_dotp_mulcomp/2
  mul_cfblk16_dotp_mulcomp/1 -> out1/1

== system gm_sampleModel12940_sub/Subsystem/cfblk173 ==
  u : Inport  OutDataTypeStr=uint8  SampleTime=1
  FixPt Constant : Constant  DisableCoverage=on  OutDataTypeStr=Inherit: Inherit via back propagation  SampleTime=-1
  FixPt Data Type Duplicate : DataTypeDuplicate  DisableCoverage=on  NumInputPorts=3
  FixPt Sum1 : Sum  OutDataTypeStr=Inherit: Inherit via back propagation  InputSameDT=on  LockScale=on
  y : Outport  SampleTime=1
  wires:
  u/1 -> FixPt Sum1/1, FixPt Data Type Duplicate/2
  FixPt Constant/1 -> FixPt Sum1/2, FixPt Data Type Duplicate/3
  FixPt Sum1/1 -> FixPt Data Type Duplicate/1, y/1

== system gm_sampleModel12940_sub/Subsystem/cfblk18 ==
  u : Inport  OutDataTypeStr=uint8  SampleTime=1
  FixPt Constant : Constant  DisableCoverage=on  OutDataTypeStr=Inherit: Inherit via back propagation  SampleTime=-1
  FixPt Data Type Duplicate : DataTypeDuplicate  DisableCoverage=on  NumInputPorts=3
  FixPt Sum1 : Sum  OutDataTypeStr=Inherit: Inherit via back propagation  InputSameDT=on  LockScale=on
  y : Outport  SampleTime=1
  wires:
  u/1 -> FixPt Sum1/1, FixPt Data Type Duplicate/2
  FixPt Constant/1 -> FixPt Sum1/2, FixPt Data Type Duplicate/3
  FixPt Sum1/1 -> FixPt Data Type Duplicate/1, y/1

== system gm_sampleModel12940_sub/Subsystem/cfblk19_inst ==
  in1 : Inport  OutDataTypeStr=uint8  SampleTime=1
  in2 : Inport  Port=2  OutDataTypeStr=uint8  SampleTime=1
  mul_cfblk19_dotp_mulcomp : Product  Inputs=**  OutDataTypeStr=uint8  SampleTime=1
  out1 : Outport  OutDataTypeStr=uint8  SampleTime=1
  wires:
  in1/1 -> mul_cfblk19_dotp_mulcomp/1
  in2/1 -> mul_cfblk19_dotp_mulcomp/2
  mul_cfblk19_dotp_mulcomp/1 -> out1/1

== system gm_sampleModel12940_sub/Subsystem/cfblk210 ==
  u : Inport  OutDataTypeStr=uint8  SampleTime=1
  FixPt Constant : Constant  DisableCoverage=on  OutDataTypeStr=Inherit: Inherit via back propagation  SampleTime=-1
  FixPt Data Type Duplicate : DataTypeDuplicate  DisableCoverage=on  NumInputPorts=3
  FixPt Sum1 : Sum  OutDataTypeStr=Inherit: Inherit via back propagation  InputSameDT=on  LockScale=on
  y : Outport  SampleTime=1
  wires:
  u/1 -> FixPt Sum1/1, FixPt Data Type Duplicate/2
  FixPt Constant/1 -> FixPt Sum1/2, FixPt Data Type Duplicate/3
  FixPt Sum1/1 -> FixPt Data Type Duplicate/1, y/1

== system gm_sampleModel12940_sub/Subsystem/cfblk212 ==
  u : Inport  OutDataTypeStr=uint8  SampleTime=1
  FixPt Constant : Constant  DisableCoverage=on  OutDataTypeStr=Inherit: Inherit via back propagation  SampleTime=-1
  FixPt Data Type Duplicate : DataTypeDuplicate  DisableCoverage=on  NumInputPorts=3
  FixPt Sum1 : Sum  OutDataTypeStr=Inherit: Inherit via back propagation  InputSameDT=on  LockScale=on
  y : Outport  SampleTime=1
  wires:
  u/1 -> FixPt Sum1/1, FixPt Data Type Duplicate/2
  FixPt Constant/1 -> FixPt Sum1/2, FixPt Data Type Duplicate/3
  FixPt Sum1/1 -> FixPt Data Type Duplicate/1, y/1

== system gm_sampleModel12940_sub/Subsystem/cfblk216_inst ==
  in1 : Inport  OutDataTypeStr=uint8  SampleTime=1
  in2 : Inport  Port=2  OutDataTypeStr=uint8  SampleTime=1
  mul_cfblk216_dotp_mulcomp : Product  Inputs=**  OutDataTypeStr=uint8  SampleTime=1
  out1 : Outport  OutDataTypeStr=uint8  SampleTime=1
  wires:
  in1/1 -> mul_cfblk216_dotp_mulcomp/1
  in2/1 -> mul_cfblk216_dotp_mulcomp/2
  mul_cfblk216_dotp_mulcomp/1 -> out1/1

== system gm_sampleModel12940_sub/Subsystem/cfblk221_inst ==
  in1 : Inport  OutDataTypeStr=uint8  SampleTime=1
  in2 : Inport  Port=2  OutDataTypeStr=uint8  SampleTime=1
  mul_cfblk221_dotp_mulcomp : Product  Inputs=**  OutDataTypeStr=uint8  SampleTime=1
  out1 : Outport  OutDataTypeStr=uint8  SampleTime=1
  wires:
  in1/1 -> mul_cfblk221_dotp_mulcomp/1
  in2/1 -> mul_cfblk221_dotp_mulcomp/2
  mul_cfblk221_dotp_mulcomp/1 -> out1/1

== system gm_sampleModel12940_sub/Subsystem/cfblk231 ==
  u : Inport  OutDataTypeStr=uint8  SampleTime=1
  FixPt Constant : Constant  DisableCoverage=on  OutDataTypeStr=Inherit: Inherit via back propagation  SampleTime=-1
  FixPt Data Type Duplicate : DataTypeDuplicate  DisableCoverage=on  NumInputPorts=3
  FixPt Sum1 : Sum  OutDataTypeStr=Inherit: Inherit via back propagation  InputSameDT=on  LockScale=on
  y : Outport  SampleTime=1
  wires:
  u/1 -> FixPt Sum1/1, FixPt Data Type Duplicate/2
  FixPt Constant/1 -> FixPt Sum1/2, FixPt Data Type Duplicate/3
  FixPt Sum1/1 -> FixPt Data Type Duplicate/1, y/1

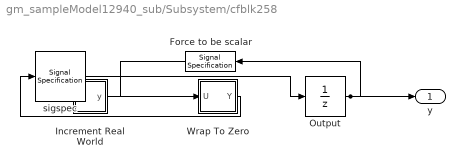
== system gm_sampleModel12940_sub/Subsystem/cfblk258 ==
  Force to be scalar : SignalSpecification  DisableCoverage=on  Dimensions=1
  Increment Real World : Subsystem  mask(Real World Value Increment){}
      mask help: Simulink:masks:RealWorldValueIncrement_MD
      mask Display: disp('V++')
  Output : UnitDelay  InitialCondition=0.0  SampleTime=tsamp  HasFrameUpgradeWarning=on
  Wrap To Zero : Subsystem  mask(Wrap To Zero){Threshold=double(7)}
      mask prompts: Threshold "Simulink:masks:Threshold_MP"
      mask help: Simulink:masks:WrapToZero_MD
  sigspec : SignalSpecification  OutDataTypeStr=uint8  Dimensions=1
  y : Outport  SampleTime=1
  wires:
  Force to be scalar/1 -> Increment Real World/1(u)
  Increment Real World/1(y) -> Wrap To Zero/1(U)
  Output/1 -> Force to be scalar/1, y/1
  Wrap To Zero/1(Y) -> sigspec/1
  sigspec/1 -> Output/1

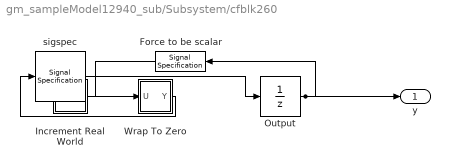
== system gm_sampleModel12940_sub/Subsystem/cfblk260 ==
  Force to be scalar : SignalSpecification  DisableCoverage=on  Dimensions=1
  Increment Real World : Subsystem  mask(Real World Value Increment){}
      mask help: Simulink:masks:RealWorldValueIncrement_MD
      mask Display: disp('V++')
  Output : UnitDelay  InitialCondition=0.0  SampleTime=tsamp  HasFrameUpgradeWarning=on
  Wrap To Zero : Subsystem  mask(Wrap To Zero){Threshold=double(65535)}
      mask prompts: Threshold "Simulink:masks:Threshold_MP"
      mask help: Simulink:masks:WrapToZero_MD
  sigspec : SignalSpecification  OutDataTypeStr=uint16  Dimensions=1
  y : Outport  SampleTime=1
  wires:
  Force to be scalar/1 -> Increment Real World/1(u)
  Increment Real World/1(y) -> Wrap To Zero/1(U)
  Output/1 -> Force to be scalar/1, y/1
  Wrap To Zero/1(Y) -> sigspec/1
  sigspec/1 -> Output/1

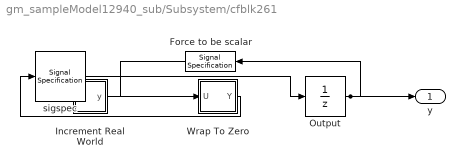
== system gm_sampleModel12940_sub/Subsystem/cfblk261 ==
  Force to be scalar : SignalSpecification  DisableCoverage=on  Dimensions=1
  Increment Real World : Subsystem  mask(Real World Value Increment){}
      mask help: Simulink:masks:RealWorldValueIncrement_MD
      mask Display: disp('V++')
  Output : UnitDelay  InitialCondition=0.0  SampleTime=tsamp  HasFrameUpgradeWarning=on
  Wrap To Zero : Subsystem  mask(Wrap To Zero){Threshold=double(7)}
      mask prompts: Threshold "Simulink:masks:Threshold_MP"
      mask help: Simulink:masks:WrapToZero_MD
  sigspec : SignalSpecification  OutDataTypeStr=uint8  Dimensions=1
  y : Outport  SampleTime=1
  wires:
  Force to be scalar/1 -> Increment Real World/1(u)
  Increment Real World/1(y) -> Wrap To Zero/1(U)
  Output/1 -> Force to be scalar/1, y/1
  Wrap To Zero/1(Y) -> sigspec/1
  sigspec/1 -> Output/1

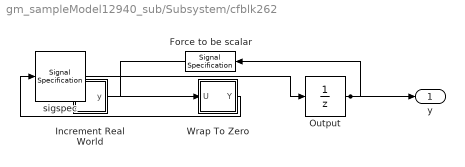
== system gm_sampleModel12940_sub/Subsystem/cfblk262 ==
  Force to be scalar : SignalSpecification  DisableCoverage=on  Dimensions=1
  Increment Real World : Subsystem  mask(Real World Value Increment){}
      mask help: Simulink:masks:RealWorldValueIncrement_MD
      mask Display: disp('V++')
  Output : UnitDelay  InitialCondition=0.0  SampleTime=tsamp  HasFrameUpgradeWarning=on
  Wrap To Zero : Subsystem  mask(Wrap To Zero){Threshold=double(7)}
      mask prompts: Threshold "Simulink:masks:Threshold_MP"
      mask help: Simulink:masks:WrapToZero_MD
  sigspec : SignalSpecification  OutDataTypeStr=uint8  Dimensions=1
  y : Outport  SampleTime=1
  wires:
  Force to be scalar/1 -> Increment Real World/1(u)
  Increment Real World/1(y) -> Wrap To Zero/1(U)
  Output/1 -> Force to be scalar/1, y/1
  Wrap To Zero/1(Y) -> sigspec/1
  sigspec/1 -> Output/1

== system gm_sampleModel12940_sub/Subsystem/cfblk263 ==
  In1 : Inport  OutDataTypeStr=uint8  PortDimensions=1  SampleTime=1
  Out1 : Outport  SampleTime=1
  wires:
  In1/1 -> Out1/1

== system gm_sampleModel12940_sub/Subsystem/cfblk264 ==
  In1 : Inport  OutDataTypeStr=uint8  PortDimensions=1  SampleTime=1
  Out1 : Outport  SampleTime=1
  wires:
  In1/1 -> Out1/1

== system gm_sampleModel12940_sub/Subsystem/cfblk265 ==
  In1 : Inport  OutDataTypeStr=uint8  PortDimensions=1  SampleTime=1
  Out1 : Outport  SampleTime=1
  wires:
  In1/1 -> Out1/1

== system gm_sampleModel12940_sub/Subsystem/cfblk266 ==
  In1 : Inport  OutDataTypeStr=uint8  PortDimensions=1  SampleTime=1
  Out1 : Outport  SampleTime=1
  wires:
  In1/1 -> Out1/1

== system gm_sampleModel12940_sub/Subsystem/cfblk267 ==
  In1 : Inport  OutDataTypeStr=uint8  PortDimensions=1  SampleTime=1
  Out1 : Outport  SampleTime=1
  wires:
  In1/1 -> Out1/1

== system gm_sampleModel12940_sub/Subsystem/cfblk269 ==
  In1 : Inport  OutDataTypeStr=uint8  PortDimensions=1  SampleTime=1
  Out1 : Outport  SampleTime=1
  wires:
  In1/1 -> Out1/1

== system gm_sampleModel12940_sub/Subsystem/cfblk270 ==
  In1 : Inport  OutDataTypeStr=uint8  PortDimensions=1  SampleTime=1
  Out1 : Outport  SampleTime=1
  wires:
  In1/1 -> Out1/1

== system gm_sampleModel12940_sub/Subsystem/cfblk3 ==
  note: U(k)
  note: Edge
  U : Inport  OutDataTypeStr=uint8  SampleTime=1
  Delay Input1 : UnitDelay  Description=Store in Global RAM  DisableCoverage=on  InitialCondition=vinit  SampleTime=-1  HasFrameUpgradeWarning=on
  FixPt Relational Operator : RelationalOperator  Operator=>  OutDataTypeStr=fixdt(0, 8)  ZeroCross=off  InputSameDT=off
  Nonpositive : Subsystem  mask(Compare To Zero){relop=<=, OutDataTypeStr=boolean, ZeroCross=off}
      mask prompts: relop "Simulink:masks:Operator_MP"; OutDataTypeStr "Simulink:masks:OutputDataType_MP"; ZeroCross "Simulink:masks:EnableZerocrossingDetection_MP"
      mask help: Simulink:masks:CompareToZero_MD
      mask init:
      | OutDataTypeStr = 'boolean';
      | ZeroCross = 'off';
      | blkName = 'sampleModel12940_sub/Subsystem/cfblk3/Nonpositive';
      | relop = '<=';
      | setValue = 'boolean';
      mask TypeOptions relop: == | ~= | < | <= | >= | >
      mask TypeOptions OutDataTypeStr: Simulink:masks:uint8 | Simulink:masks:boolean
      mask Callback ZeroCross: sl('zeroCrossEnable', gcbh);
      mask Display: disp([relop,' 0'])
  Y : Outport  SampleTime=1
  wires:
  U/1 -> Nonpositive/1(u)
  Delay Input1/1 -> FixPt Relational Operator/2
  FixPt Relational Operator/1 -> Y/1
  Nonpositive/1(y) -> FixPt Relational Operator/1, Delay Input1/1

== system gm_sampleModel12940_sub/Subsystem/cfblk31 ==
  u : Inport  OutDataTypeStr=uint8  SampleTime=1
  FixPt Constant : Constant  DisableCoverage=on  OutDataTypeStr=Inherit: Inherit via back propagation  SampleTime=-1
  FixPt Data Type Duplicate : DataTypeDuplicate  DisableCoverage=on  NumInputPorts=3
  FixPt Sum1 : Sum  OutDataTypeStr=Inherit: Inherit via back propagation  InputSameDT=on  LockScale=on
  y : Outport  SampleTime=1
  wires:
  u/1 -> FixPt Sum1/1, FixPt Data Type Duplicate/2
  FixPt Constant/1 -> FixPt Sum1/2, FixPt Data Type Duplicate/3
  FixPt Sum1/1 -> FixPt Data Type Duplicate/1, y/1

== system gm_sampleModel12940_sub/Subsystem/cfblk35 ==
  u : Inport  OutDataTypeStr=uint8  SampleTime=1
  FixPt Constant : Constant  DisableCoverage=on  OutDataTypeStr=Inherit: Inherit via back propagation  SampleTime=-1
  FixPt Data Type Duplicate : DataTypeDuplicate  DisableCoverage=on  NumInputPorts=3
  FixPt Sum1 : Sum  OutDataTypeStr=Inherit: Inherit via back propagation  InputSameDT=on  LockScale=on
  y : Outport  SampleTime=1
  wires:
  u/1 -> FixPt Sum1/1, FixPt Data Type Duplicate/2
  FixPt Constant/1 -> FixPt Sum1/2, FixPt Data Type Duplicate/3
  FixPt Sum1/1 -> FixPt Data Type Duplicate/1, y/1

== system gm_sampleModel12940_sub/Subsystem/cfblk36 ==
  u : Inport  OutDataTypeStr=uint8  SampleTime=1
  FixPt Constant : Constant  DisableCoverage=on  OutDataTypeStr=Inherit: Inherit via back propagation  SampleTime=-1
  FixPt Data Type Duplicate : DataTypeDuplicate  DisableCoverage=on  NumInputPorts=3
  FixPt Sum1 : Sum  OutDataTypeStr=Inherit: Inherit via back propagation  InputSameDT=on  LockScale=on
  y : Outport  SampleTime=1
  wires:
  u/1 -> FixPt Sum1/1, FixPt Data Type Duplicate/2
  FixPt Constant/1 -> FixPt Sum1/2, FixPt Data Type Duplicate/3
  FixPt Sum1/1 -> FixPt Data Type Duplicate/1, y/1

== system gm_sampleModel12940_sub/Subsystem/cfblk47 ==
  u : Inport  OutDataTypeStr=uint8  SampleTime=1
  FixPt Constant : Constant  DisableCoverage=on  OutDataTypeStr=Inherit: Inherit via back propagation  SampleTime=-1
  FixPt Data Type Duplicate : DataTypeDuplicate  DisableCoverage=on  NumInputPorts=3
  FixPt Sum1 : Sum  OutDataTypeStr=Inherit: Inherit via back propagation  InputSameDT=on  LockScale=on
  y : Outport  SampleTime=1
  wires:
  u/1 -> FixPt Sum1/1, FixPt Data Type Duplicate/2
  FixPt Constant/1 -> FixPt Sum1/2, FixPt Data Type Duplicate/3
  FixPt Sum1/1 -> FixPt Data Type Duplicate/1, y/1

== system gm_sampleModel12940_sub/Subsystem/cfblk57 ==
  u : Inport  OutDataTypeStr=uint8  SampleTime=1
  FixPt Constant : Constant  DisableCoverage=on  OutDataTypeStr=Inherit: Inherit via back propagation  SampleTime=-1
  FixPt Data Type Duplicate : DataTypeDuplicate  DisableCoverage=on  NumInputPorts=3
  FixPt Sum1 : Sum  OutDataTypeStr=Inherit: Inherit via back propagation  InputSameDT=on  LockScale=on
  y : Outport  SampleTime=1
  wires:
  u/1 -> FixPt Sum1/1, FixPt Data Type Duplicate/2
  FixPt Constant/1 -> FixPt Sum1/2, FixPt Data Type Duplicate/3
  FixPt Sum1/1 -> FixPt Data Type Duplicate/1, y/1

== system gm_sampleModel12940_sub/Subsystem/cfblk63_inst ==
  in1 : Inport  OutDataTypeStr=uint8  SampleTime=1
  in2 : Inport  Port=2  OutDataTypeStr=uint8  SampleTime=1
  mul_cfblk63_dotp_mulcomp : Product  Inputs=**  OutDataTypeStr=uint8  SampleTime=1
  out1 : Outport  OutDataTypeStr=uint8  SampleTime=1
  wires:
  in1/1 -> mul_cfblk63_dotp_mulcomp/1
  in2/1 -> mul_cfblk63_dotp_mulcomp/2
  mul_cfblk63_dotp_mulcomp/1 -> out1/1

== system gm_sampleModel12940_sub/Subsystem/cfblk78_inst ==
  in1 : Inport  OutDataTypeStr=uint8  SampleTime=1
  in2 : Inport  Port=2  OutDataTypeStr=uint8  SampleTime=1
  mul_cfblk78_dotp_mulcomp : Product  Inputs=**  OutDataTypeStr=uint8  SampleTime=1
  out1 : Outport  OutDataTypeStr=uint8  SampleTime=1
  wires:
  in1/1 -> mul_cfblk78_dotp_mulcomp/1
  in2/1 -> mul_cfblk78_dotp_mulcomp/2
  mul_cfblk78_dotp_mulcomp/1 -> out1/1

== system gm_sampleModel12940_sub/Subsystem/cfblk81_inst ==
  in1 : Inport  OutDataTypeStr=uint8  SampleTime=1
  in2 : Inport  Port=2  OutDataTypeStr=uint8  SampleTime=1
  mul_cfblk81_dotp_mulcomp : Product  Inputs=**  OutDataTypeStr=uint8  SampleTime=1
  out1 : Outport  OutDataTypeStr=uint8  SampleTime=1
  wires:
  in1/1 -> mul_cfblk81_dotp_mulcomp/1
  in2/1 -> mul_cfblk81_dotp_mulcomp/2
  mul_cfblk81_dotp_mulcomp/1 -> out1/1

== system gm_sampleModel12940_sub/Subsystem/cfblk84 ==
  u : Inport  OutDataTypeStr=uint8  SampleTime=1
  FixPt Constant : Constant  DisableCoverage=on  OutDataTypeStr=Inherit: Inherit via back propagation  SampleTime=-1
  FixPt Data Type Duplicate : DataTypeDuplicate  DisableCoverage=on  NumInputPorts=3
  FixPt Sum1 : Sum  OutDataTypeStr=Inherit: Inherit via back propagation  InputSameDT=on  LockScale=on
  y : Outport  SampleTime=1
  wires:
  u/1 -> FixPt Sum1/1, FixPt Data Type Duplicate/2
  FixPt Constant/1 -> FixPt Sum1/2, FixPt Data Type Duplicate/3
  FixPt Sum1/1 -> FixPt Data Type Duplicate/1, y/1

== system gm_sampleModel12940_sub/Subsystem/cfblk94_inst ==
  in1 : Inport  OutDataTypeStr=uint8  SampleTime=1
  in2 : Inport  Port=2  OutDataTypeStr=uint8  SampleTime=1
  mul_cfblk94_dotp_mulcomp : Product  Inputs=**  OutDataTypeStr=uint8  SampleTime=1
  out1 : Outport  OutDataTypeStr=uint8  SampleTime=1
  wires:
  in1/1 -> mul_cfblk94_dotp_mulcomp/1
  in2/1 -> mul_cfblk94_dotp_mulcomp/2
  mul_cfblk94_dotp_mulcomp/1 -> out1/1

== system gm_sampleModel12940_sub/Subsystem/cfblk98 ==
  u : Inport  OutDataTypeStr=uint8  SampleTime=1
  FixPt Constant : Constant  DisableCoverage=on  OutDataTypeStr=Inherit: Inherit via back propagation  SampleTime=-1
  FixPt Data Type Duplicate : DataTypeDuplicate  DisableCoverage=on  NumInputPorts=3
  FixPt Sum1 : Sum  OutDataTypeStr=Inherit: Inherit via back propagation  InputSameDT=on  LockScale=on
  y : Outport  SampleTime=1
  wires:
  u/1 -> FixPt Sum1/1, FixPt Data Type Duplicate/2
  FixPt Constant/1 -> FixPt Sum1/2, FixPt Data Type Duplicate/3
  FixPt Sum1/1 -> FixPt Data Type Duplicate/1, y/1

== system gm_sampleModel12940_sub/Subsystem/cfblk12/Positive ==
  u : Inport  OutDataTypeStr=uint8  SampleTime=1
  Compare : RelationalOperator  Operator=>  OutDataTypeStr=boolean  ZeroCross=off
  Constant : Constant  DisableCoverage=on  Value=0  OutDataTypeStr=Inherit: Inherit via back propagation  SampleTime=-1  PreserveConstantTs=on
  y : Outport  SampleTime=1
  wires:
  u/1 -> Compare/1
  Compare/1 -> y/1
  Constant/1 -> Compare/2

== system gm_sampleModel12940_sub/Subsystem/cfblk258/Increment Real World ==
  u : Inport  OutDataTypeStr=uint8  SampleTime=1
  FixPt Constant : Constant  DisableCoverage=on  OutDataTypeStr=Inherit: Inherit via back propagation  SampleTime=-1
  FixPt Data Type Duplicate : DataTypeDuplicate  DisableCoverage=on  NumInputPorts=3
  FixPt Sum1 : Sum  OutDataTypeStr=Inherit: Inherit via back propagation  InputSameDT=on  LockScale=on
  y : Outport  SampleTime=1
  wires:
  u/1 -> FixPt Sum1/1, FixPt Data Type Duplicate/2
  FixPt Constant/1 -> FixPt Sum1/2, FixPt Data Type Duplicate/3
  FixPt Sum1/1 -> FixPt Data Type Duplicate/1, y/1

== system gm_sampleModel12940_sub/Subsystem/cfblk258/Wrap To Zero ==
  note: U(k)
  U : Inport  OutDataTypeStr=uint8  SampleTime=1
  Constant : Constant  DisableCoverage=on  Value=0  OutDataTypeStr=Inherit: Inherit via back propagation  SampleTime=-1
  FixPt Data Type Duplicate1 : DataTypeDuplicate  DisableCoverage=on  NumInputPorts=3
  FixPt Switch : Switch  Criteria=u2 > Threshold  Threshold=Threshold  OutDataTypeStr=Inherit: Inherit via back propagation  ZeroCross=off  SaturateOnIntegerOverflow=off  InputSameDT=off
  Y : Outport  SampleTime=1
  wires:
  U/1 -> FixPt Switch/3, FixPt Switch/2, FixPt Data Type Duplicate1/2
  Constant/1 -> FixPt Switch/1, FixPt Data Type Duplicate1/3
  FixPt Switch/1 -> FixPt Data Type Duplicate1/1, Y/1

== system gm_sampleModel12940_sub/Subsystem/cfblk260/Increment Real World ==
  u : Inport  OutDataTypeStr=uint16  SampleTime=1
  FixPt Constant : Constant  DisableCoverage=on  OutDataTypeStr=Inherit: Inherit via back propagation  SampleTime=-1
  FixPt Data Type Duplicate : DataTypeDuplicate  DisableCoverage=on  NumInputPorts=3
  FixPt Sum1 : Sum  OutDataTypeStr=Inherit: Inherit via back propagation  InputSameDT=on  LockScale=on
  y : Outport  SampleTime=1
  wires:
  u/1 -> FixPt Sum1/1, FixPt Data Type Duplicate/2
  FixPt Constant/1 -> FixPt Sum1/2, FixPt Data Type Duplicate/3
  FixPt Sum1/1 -> FixPt Data Type Duplicate/1, y/1

== system gm_sampleModel12940_sub/Subsystem/cfblk260/Wrap To Zero ==
  note: U(k)
  U : Inport  OutDataTypeStr=uint16  SampleTime=1
  Constant : Constant  DisableCoverage=on  Value=0  OutDataTypeStr=Inherit: Inherit via back propagation  SampleTime=-1
  FixPt Data Type Duplicate1 : DataTypeDuplicate  DisableCoverage=on  NumInputPorts=3
  FixPt Switch : Switch  Criteria=u2 > Threshold  Threshold=Threshold  OutDataTypeStr=Inherit: Inherit via back propagation  ZeroCross=off  SaturateOnIntegerOverflow=off  InputSameDT=off
  Y : Outport  SampleTime=1
  wires:
  U/1 -> FixPt Switch/3, FixPt Switch/2, FixPt Data Type Duplicate1/2
  Constant/1 -> FixPt Switch/1, FixPt Data Type Duplicate1/3
  FixPt Switch/1 -> FixPt Data Type Duplicate1/1, Y/1
